simulink model "ElectricalID_ref"  (R2022b)
settings: Solver=FixedStepDiscrete  StartTime=0.0  StopTime=160  FixedStep=0.000005  RelTol=1e-3  EnableMultiTasking=on
settings Model: RequirementInfo={} %GIDa_fe9045fd_0412_4b6e_8206_617cc20e6fde  FPTRunName=Active  Creator=ts  LastModifiedBy=hufnagelde
settings SolverCC: AlgebraicLoopSolver=TrustRegion  PositivePriorityOrder=on  AutoInsertRateTranBlk=on
settings DataIOCC: SaveOutput=off  SignalLogging=off  DSMLogging=off  SaveTime=off
settings OptimizationCC: DefaultParameterBehavior=Inlined  UseDivisionForNetSlopeComputation=on  GainParamInheritBuiltInType=on  UseFloatMulNetSlope=on  DefaultUnderspecifiedDataType=single  UseSpecifiedMinMax=on  InlineInvariantSignals=on  PassReuseOutputArgsAs=Individual arguments  ZeroExternalMemoryAtStartup=off  ZeroInternalMemoryAtStartup=off  NoFixptDivByZeroProtection=on  EfficientFloat2IntCast=on  LifeSpan=1  MaxStackSize=64  OptimizeBlockOrder=speed  DifferentSizesBufferReuse=on  EfficientTunableParamExpr=on
settings DebuggingCC: UnconnectedInputMsg=warning  UnconnectedOutputMsg=warning  UnconnectedLineMsg=warning  BusObjectLabelMismatch=error  AllowSymbolicDim=off  SFUnexpectedBacktrackingDiag=warning  SFNoUnconditionalDefaultTransitionDiag=warning  SFExecutionAtInitializationDiag=none  SFMachineParentedDataDiag=warning  ArithmeticOperatorsInVariantConditions=warning
settings HardwareCC: ProdBitPerPointer=32  ProdBitPerSizeT=32  ProdBitPerPtrDiffT=32  ProdLargestAtomicInteger=Long  ProdLargestAtomicFloat=Double  ProdWordSize=32  ProdLongLongMode=on  ProdHWDeviceType=ARM Compatible->ARM Cortex-R  HardwareBoardFeatureSet=SoCBlockset
settings ModelReferenceCC: EnableRefExpFcnMdlSchedulingChecks=on
settings SFSimCC: SimGenImportedTypeDefs=on  MATLABDynamicMemAlloc=off
settings RTWCC: Description=Embedded Coder  SystemTargetFile=ert.tlc  GenCodeOnly=on  TemplateMakefile=ert_default_tmf  GenerateReport=on  BuildConfiguration=Faster Runs  IncludeHyperlinkInReport=on  LaunchReport=on  GenerateTraceInfo=on  GenerateTraceReport=on  GenerateTraceReportSl=on  GenerateTraceReportSf=on  GenerateTraceReportEml=on  GenerateCodeMetricsReport=on  CheckMdlBeforeBuild=Warning  DLArmComputeVersion=19.05
settings CodeAppCC: ForceParamTrailComments=on  IgnoreCustomStorageClasses=off  OperatorAnnotations=on  SimulinkDataObjDesc=on  SFDataObjDesc=on  MATLABFcnDesc=on  CustomSymbolStrGlobalVar=rt$M$R$N  CustomSymbolStrType=$N$M$R_t  CustomSymbolStrFcn=$N$M$F  CustomSymbolStrMacro=$N$M  InsertBlockDesc=on  StateflowObjectComments=on  MATLABSourceComments=on  EnableCustomComments=on  ReqsInCode=on
settings ERTTargetCC: TargetLangStandard=C99 (ISO)  CodeReplacementLibrary=GNU C99 extensions  MultiwordLength=2048  IncludeMdlTerminateFcn=off  CombineSignalStateStructs=on  SuppressErrorStatus=on  IncludeFileDelimiter=UseQuote  SupportAbsoluteTime=off  CodeInterfacePackaging=Reusable function  SupportNonFinite=off  RemoveResetFunc=off  InlinedParameterPlacement=NonHierarchical  MultiInstanceErrorCode=Warning  RootIOFormat=Part of model data structure  ERTCustomFileTemplate=example_file_process.tlc  GlobalDataDefinition=InSourceFile  GlobalDataReference=InSourceFile  ERTFilePackagingFormat=CompactWithDataFile  SuppressUnreachableDefaultCases=off
settings ConfigComp: CovScope=ReferencedModels  CovSaveName=covdata_rollAP  CovMetricSettings=dcmtrwe  CovHTMLOptions=-sRT=1 -aTS=1 -bRG=1 -bTC=1 -hTR=1 -nFC=0 -scm=1 -bcm=1 -xEv=0  CovSaveCumulativeToWorkspaceVar=on  CovSaveSingleToWorkspaceVar=on  CovCumulativeVarName=covCumulativeData_rollAP  CovReportOnPause=off  CovExternalEMLEnable=off  CovSFcnEnable=off

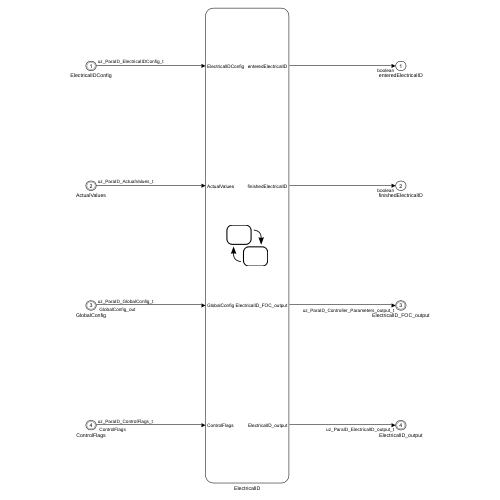
[thumbnail: Simulink's stored preview of the top-level diagram]
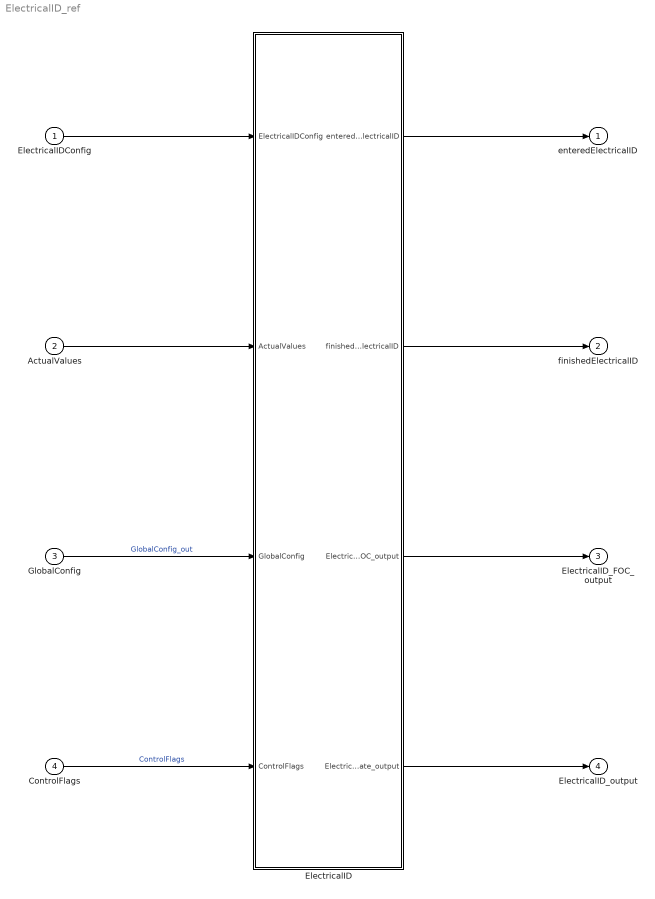
== system ElectricalID_ref ==
  ElectricalIDConfig : Inport  OutDataTypeStr=Bus: uz_ParaID_ElectricalIDConfig_t  PortDimensions=1  SampleTime=[5.0000000000000002e-05,0]  BusOutputAsStruct=on
  ActualValues : Inport  Port=2  OutDataTypeStr=Bus: uz_ParaID_ActualValues_t  PortDimensions=1  SampleTime=[5.0000000000000002e-05,0]  BusOutputAsStruct=on
  GlobalConfig : Inport  Port=3  OutDataTypeStr=Bus: uz_ParaID_GlobalConfig_t  PortDimensions=1  SampleTime=[5.0000000000000002e-05,0]  BusOutputAsStruct=on
  ControlFlags : Inport  Port=4  OutDataTypeStr=Bus: uz_ParaID_ControlFlags_t  PortDimensions=1  SampleTime=[5.0000000000000002e-05,0]  BusOutputAsStruct=on
  ElectricalID : Stateflow chart
  enteredElectricalID : Outport  OutDataTypeStr=boolean  PortDimensions=1  SampleTime=[5.0000000000000002e-05,0]
  finishedElectricalID : Outport  Port=2  OutDataTypeStr=boolean  PortDimensions=1  SampleTime=[5.0000000000000002e-05,0]
  ElectricalID_FOC_output : Outport  Port=3  OutDataTypeStr=Bus: uz_ParaID_Controller_Parameters_output_t  PortDimensions=1  SampleTime=[5.0000000000000002e-05,0]  BusOutputAsStruct=on
  ElectricalID_output : Outport  Port=4  OutDataTypeStr=Bus: uz_ParaID_ElectricalID_output_t  PortDimensions=1  SampleTime=[5.0000000000000002e-05,0]  BusOutputAsStruct=on
  wires:
  ElectricalIDConfig/1 -> ElectricalID/1(ElectricalIDConfig)
  ActualValues/1 -> ElectricalID/2(ActualValues)
  GlobalConfig/1 -> ElectricalID/3(GlobalConfig)  "GlobalConfig_out"
  ControlFlags/1 -> ElectricalID/4(ControlFlags)  "ControlFlags"
  ElectricalID/1(enteredElectricalID) -> enteredElectricalID/1
  ElectricalID/2(finishedElectricalID) -> finishedElectricalID/1
  ElectricalID/3(ElectricalID_FOC_output) -> ElectricalID_FOC_output/1
  ElectricalID/4(ElectricalID_state_output) -> ElectricalID_output/1

== stateflow chart ElectricalID_ref/ElectricalID ==
  settings: updateMethod=DISCRETE  sampleTime=1/d_f_states
  note: PMSM identification
  state ElectricalID
    entry:
    initParams;
    ElectricalID_FOC_output.activeState = uint16(100);
    enteredElectricalID=boolean(1);
    during:
    state stepResponse_q
      entry:
      ElectricalID_FOC_output.activeState = uint16(142);
      resetParams_LM;
      z = uint16(1);
      ElectricalID_state_output.enable_TriState          = [boolean(1),boolean(0),boolean(0)];
      ElectricalID_state_output.PWM_Switch_0 = single(0);
      counter = uint32(1);
      during:
      ElectricalID_state_output.PWM_Switch_4 = single(DutyCycle);
      if(counter <= 1024)
      if(counter > 1)
      measArray1(counter-1) = ActualValues.I_abc.c;
      if(mod(counter,5) == 0)
      Vstep(z-1) = ActualValues.V_abc.b+ActualValues.V_abc.c;
      z = z + 1;
      end
      counter = counter + 1;
      end
      if(counter == 1)
      counter = counter + 1;
      Vstep(1) = ActualValues.V_abc.c+ActualValues.V_abc.b;
      z = z + 1;
      end
      else
      if(counter == 1025)
      measArray1(counter-1) = ActualValues.I_abc.c;
      Vstep(z-1) = ActualValues.V_abc.b+ActualValues.V_abc.c;
      V0 = mean(Vstep);
      end
      ElectricalID_state_output.PWM_Switch_4 = single(0);
      counter = counter + 1;
      end
      exit:
      ElectricalID_state_output.enable_TriState          = [boolean(0),boolean(0),boolean(0)];
    state evaluate_Turn_DC
      entry:
      ElectricalID_FOC_output.activeState = uint16(110);
      counter = uint32(1);
      omega_register=single(zeros(5,1));
      if(ElectricalIDConfig.dutyCyc > 0.0) %Checks if a manual value for the DutyCycle was set
      DutyCycle = single(ElectricalIDConfig.dutyCyc);
      DC_manual = boolean(1);
      else
      DutyCycle = single(0.01);
      end
      during:
      if(DC_manual == 0); %averages the last 0.1s
      omega_sum=omega_sum+single(ActualValues.omega_m);
      if(mod(counter,uint32(0.1/GlobalConfig.sampleTimeISR))==0)
      RefreshDataRegister;
      omega_register(1,1)=omega_sum*(GlobalConfig.sampleTimeISR/0.1);
      omega_sum=single(0);
      end
      if(mod(counter,uint32(2/GlobalConfig.sampleTimeISR))==0)%after 2s omega will be evaluated
      DutyCycle_mod(abs(omega_register));
      end
      end
      counter = counter + 1;
      TurnMotor;
      exit:
      ElectricalID_state_output.PWM_Switch_0 = single(0);
      ElectricalID_state_output.PWM_Switch_2 = single(0);
      ElectricalID_state_output.PWM_Switch_4 = single(0);
    state alignRotor_d_off2
      entry:counter = uint32(1);
      ElectricalID_FOC_output.activeState = uint16(131);
      during:counter = counter +1;
      exit:
    state measure_psiPM
      entry:
      ElectricalID_FOC_output.activeState = uint16(150);
      ElectricalID_FOC_output.enableFOC_speed = boolean(1);
      ElectricalID_FOC_output.n_ref_FOC = ElectricalIDConfig.n_ref_measurement;
      wait_count = uint32(3/GlobalConfig.sampleTimeISR);
      during:
      if(counter > wait_count && counter < (wait_count+1025))
      measArray1(counter-wait_count) = ActualValues.v_dq.q;
      d(counter-wait_count) = ActualValues.i_dq.q;
      i_est(counter-wait_count) = ActualValues.omega_el;
      end
      if(counter == (wait_count+1025))
      ElectricalID_state_output.PMSM_parameters.Psi_PM_Vs = (mean(measArray1(1:1024))-mean(d(1:1024))*....
      ElectricalID_state_output.PMSM_parameters.R_ph_Ohm)/(mean(i_est(1:1024)));
      end
      counter = counter + 1;
      exit:
      counter = uint32(1);
    state stepResponse		%state 2.0
      entry:
      ElectricalID_FOC_output.activeState = uint16(140);
      counter = uint32(1);
      z = uint16(1);
      during:
      ElectricalID_state_output.PWM_Switch_0 = single(DutyCycle);
      if(counter <= 1024)
      if(counter > 1)
      measArray1(counter-1) = ActualValues.I_abc.a;
      if(mod(counter,5) == 0)
      Vstep(z-1) = ActualValues.V_abc.a;
      z = z + 1;
      end
      counter = counter + 1;
      end
      if(counter == 1)
      counter = counter + 1
      Vstep(1) = ActualValues.V_abc.a;
      z = z + 1;
      end
      else
      if(counter == 1025)
      measArray1(counter-1) = ActualValues.I_abc.a;
      Vstep(z-1) = ActualValues.I_abc.a;
      V0 = mean(Vstep);
      end
      ElectricalID_state_output.PWM_Switch_0 = single(0);
      counter = counter + 1;
      end
      exit:
      ElectricalID_FOC_output.activeState = uint16(22);
    state stop 	%state 10.1
      entry:
      ElectricalID_FOC_output.activeState = uint16(151);
      ElectricalID_FOC_output.n_ref_FOC = single(0);
      ElectricalID_FOC_output.resetIntegrator = boolean(1);
      during:counter = counter +1;
    state rotorInertiaEstimation
      entry:
      ElectricalID_FOC_output.enableFOC_speed = boolean(0);
      ElectricalID_FOC_output.enableFOC_torque = boolean(1);
      counter = uint32(1);
      ElectricalID_FOC_output.resetIntegrator = boolean(0);
      ElectricalID_FOC_output.activeState = uint16(160);
      wait_count = uint32(3/GlobalConfig.sampleTimeISR);
      during:
      ElectricalID_FOC_output.M_ref_FOC = SinusGenerator(ElectricalIDConfig.goertzlTorque,....
      ElectricalIDConfig.goertzlFreq,GlobalConfig.sampleTimeISR);
      if(counter > wait_count && counter < (wait_count+501))
      measArray1(counter-wait_count) = ActualValues.i_dq.q;
      i_est(counter-wait_count) = ActualValues.omega_m;
      end
      counter = counter + 1;
      exit:
      goertzel;
    state alignRotor_d_on
      entry:
      ElectricalID_FOC_output.activeState = uint16(120);
      counter = uint32(1);
      during:
      DutyCycle_filt = single(single(counter)*GlobalConfig.sampleTimeISR*2);
      if(DutyCycle_filt > 1)
      DutyCycle_filt = single(1.0);
      end
      ElectricalID_state_output.PWM_Switch_0 = single(DutyCycle*DutyCycle_filt);
      ElectricalID_state_output.PWM_Switch_2 = single(0);
      ElectricalID_state_output.PWM_Switch_4 = single(0);
      counter  = counter +1;
      exit:
      ElectricalID_state_output.PWM_Switch_0 = single(0);
    state Levenberg_Marquardt_q
      entry:
      ElectricalID_FOC_output.activeState = uint16(143);
      LM_algorithm_Lq;
      ElectricalID_state_output.PMSM_parameters.Lq_Henry = L_est*0.5;
      during:
      exit:
    state alignRotor_d_off
      entry:counter = uint32(1);
      ElectricalID_FOC_output.activeState = uint16(121);
      during:counter  = counter +1;
      exit:
      ElectricalID_state_output.thetaOffset = ActualValues.theta_m;
      DutyCycle=single(0.0);%resets the DC and DC_manual flag, so that for the step-response
      DC_manual=boolean(0);  %a new DC can be entered
    state endState
      entry:
      counter = uint32(1);
      ElectricalID_FOC_output.activeState = uint16(161);
      ElectricalID_FOC_output.resetIntegrator=boolean(1);
      ElectricalID_FOC_output.M_ref_FOC = single(0.0);
      during:
      counter = counter + 1;
    state Levenberg_Marquardt 		%state 3.0
      entry:
      ElectricalID_FOC_output.activeState = uint16(141);
      LM_algorithm;
      % calculate R and L. Considering that all three phases
      % are connected and that a delta connected winding has
      % to be calculated into star connected values, the factor
      % is 2/3 for delta and star connected windings.
      % Therefore Rs and Ld are the values expressed in
      % star connection
      ElectricalID_state_output.PMSM_parameters.R_ph_Ohm = (R_est-R_corr)*2.0/3.0;
      ElectricalID_state_output.PMSM_parameters.Ld_Henry = L_est*2.0/3.0;
      during:
      exit:
    state calculatePIcontroller 	%state6.0
      entry:
      ElectricalID_FOC_output.activeState = uint16(144);
      % calculation according to Gemaßmer KIT
      Kp_id_loc = ElectricalID_state_output.PMSM_parameters.Ld_Henry / (3.0 * GlobalConfig.sampleTimeISR) ;
      Ki_id_loc = ElectricalID_state_output.PMSM_parameters.R_ph_Ohm / (3.0 * GlobalConfig.sampleTimeISR) ;
      Ki_iq_loc = Ki_id_loc;
      if (ElectricalIDConfig.identLq == 1)
      Kp_iq_loc = ElectricalID_state_output.PMSM_parameters.Lq_Henry / (3.0 * GlobalConfig.sampleTimeISR) ;
      elseif (ElectricalIDConfig.identLq == 0)
      ElectricalID_state_output.PMSM_parameters.Lq_Henry = ....
      ElectricalID_state_output.PMSM_parameters.Ld_Henry;
      Kp_iq_loc = Kp_id_loc;
      end
      Kp_n_loc = Kp_iq_loc/(ElectricalID_state_output.PMSM_parameters.Lq_Henry*dampingFactor*....
      GlobalConfig.PMSM_config.polePairs*3.0/2.0*psiOverJ);
      Ki_n_loc = (Kp_iq_loc * Kp_iq_loc)/( ElectricalID_state_output.PMSM_parameters.Lq_Henry *....
      ElectricalID_state_output.PMSM_parameters.Lq_Henry  * dampingFactor * dampingFactor * ....
      dampingFactor * GlobalConfig.PMSM_config.polePairs...
      *3.0/2.0*psiOverJ);
      %Output calculated values
      ElectricalID_FOC_output.Kp_id_out = Kp_id_loc;
      ElectricalID_FOC_output.Ki_id_out = Ki_id_loc;
      ElectricalID_FOC_output.Kp_iq_out = Kp_iq_loc;
      ElectricalID_FOC_output.Ki_iq_out = Ki_iq_loc;
      ElectricalID_FOC_output.Kp_n_out = Kp_n_loc;
      ElectricalID_FOC_output.Ki_n_out = single(Ki_n_loc);
    state findDutyCycle	%Motor must be manually locked via load machine until state 60
      entry:
      ElectricalID_FOC_output.activeState = uint16(130);
      if(ElectricalIDConfig.dutyCyc > 0.0)%Checks if a manual value for the DutyCycle was set
      DutyCycle = single(ElectricalIDConfig.dutyCyc);
      DC_manual = boolean(1);
      else
      DutyCycle = single(0.005);
      end
      counter = uint32(1); %starts with 1, so that the DutyCylce_mod function wont be entered
      %during the fist cycle through the state
      during:
      if(DC_manual == 0 && ia_valid==0)
      ElectricalID_state_output.PWM_Switch_0 = single(DutyCycle);
      if(counter < uint32(0.4/GlobalConfig.sampleTimeISR))
      counter = counter +1;
      elseif(counter >= uint32(0.4/GlobalConfig.sampleTimeISR) &&....
      counter < uint32(0.5/GlobalConfig.sampleTimeISR))
      counter = counter +1;
      ia_sum=ia_sum+single(ActualValues.I_abc.a);
      elseif(counter == uint32(0.5/GlobalConfig.sampleTimeISR))
      DutyCycle_mod(abs(ia_sum*(GlobalConfig.sampleTimeISR/0.1)));
      counter  = uint32(1);
      ia_sum = single(0.0);
      end
      end
      exit:
      ElectricalID_state_output.PWM_Switch_0 = single(0);
    state waitState 	%do nothing
      entry:
      counter = uint32(1);
      ElectricalID_FOC_output.enableFOC_torque= boolean(0);
      ElectricalID_FOC_output.activeState = uint16(170);
      % recalculate speed controller using psiPM and J
      Ki_n_loc =....
      (Kp_iq_loc * Kp_iq_loc * 2.0 * pi * ElectricalID_state_output.PMSM_parameters.J_kg_m_squared) /....
      (dampingFactor * dampingFactor * dampingFactor * ElectricalID_state_output.PMSM_parameters.Lq_Henry....
      *ElectricalID_state_output.PMSM_parameters.Lq_Henry *....
      ElectricalID_state_output.PMSM_parameters.Psi_PM_Vs....
      * ElectricalID_state_output.PMSM_parameters.polePairs * 90.0);
      Kp_n_loc =....
      sqrt((dampingFactor * Ki_n_loc * 2.0 * pi * ElectricalID_state_output.PMSM_parameters.J_kg_m_squared)...
      / (90.0 * ElectricalID_state_output.PMSM_parameters.polePairs *....
      ElectricalID_state_output.PMSM_parameters.Psi_PM_Vs));
      ElectricalID_FOC_output.Kp_n_out = Kp_n_loc;
      ElectricalID_FOC_output.Ki_n_out = Ki_n_loc;
      ElectricalID_state_output.PMSM_parameters.I_max_Ampere = GlobalConfig.PMSM_config.I_max_Ampere;
      during:
      counter = counter + 1;
      exit:
      finishedElectricalID=boolean(1);
      enteredElectricalID=boolean(0);
      reset_FOC_output;
    (default) -> evaluate_Turn_DC
    calculatePIcontroller 	%state6.0 -> measure_psiPM : [GlobalConfig.ACCEPT==1]
    findDutyCycle	%Motor must be manually locked via load machine until state 60 -> alignRotor_d_off2 : [ia_valid==1 ||DC_manual == 1]
    alignRotor_d_off2 -> stepResponse		%state 2.0 : [one_sec_transition_counter == counter]
    measure_psiPM -> stop 	%state 10.1 : [ElectricalID_state_output.PMSM_parameters.Psi_PM_Vs > 0]
    stop 	%state 10.1 -> rotorInertiaEstimation : [one_sec_transition_counter == counter]
    evaluate_Turn_DC -> alignRotor_d_on [order 1] : [om_con==1]
    evaluate_Turn_DC -> alignRotor_d_on [order 2] : [DC_manual == 1]
    Levenberg_Marquardt 		%state 3.0 -> stepResponse_q [order 2] : [GlobalConfig.ACCEPT == 1 ....
        | && ElectricalIDConfig.identLq == 1]
    stepResponse_q -> Levenberg_Marquardt_q : [counter == 1026]
    alignRotor_d_on -> alignRotor_d_off : [one_sec_transition_counter == counter]
    stepResponse		%state 2.0 -> Levenberg_Marquardt 		%state 3.0 : [counter == 1026]
    rotorInertiaEstimation -> endState : [counter == (wait_count+513)]
    Levenberg_Marquardt_q -> calculatePIcontroller 	%state6.0
    alignRotor_d_off -> findDutyCycle	%Motor must be manually locked via load machine until state 60 : [one_sec_transition_counter == counter]
    endState -> waitState 	%do nothing : [one_sec_transition_counter == counter]
    Levenberg_Marquardt 		%state 3.0 -> calculatePIcontroller 	%state6.0 [order 1] : [GlobalConfig.ACCEPT == 1 &&....
        |  ElectricalIDConfig.identLq == 0]
  state Waiting
    entry:
    %wait for activation of
    %ElectricalID
    %donothing
  Waiting -> ElectricalID [order 1] : [ControlFlags.startElectricalID==1 &&....
      |  GlobalConfig.Reset==0 && GlobalConfig.ACCEPT==1]
  (default) -> Waiting
  Waiting -> Waiting [order 2] : [GlobalConfig.Reset==1]
      | {finishedElectricalID=boolean(0);
      | enteredElectricalID=boolean(0);
      | initParams;}
  waitState 	%do nothing -> Waiting : [one_sec_transition_counter == counter]
  ElectricalID -> Waiting : [GlobalConfig.Reset==1 || GlobalConfig.ElectricalID==0 ||....
      |  GlobalConfig.enableParameterID==0]
      | {enteredElectricalID=boolean(0);initParams;}
  data: om_reg_in function_input; Amp function_input; Freq function_input; sampleTime function_input; y function_output; ia_reg_in function_input; n_filt local single size=1 =single(0.0); n_ref_old local single size=1 =single(0.0); repetitionCounter local uint32 size=1 =uint32(0); dutyCycAdj local single size=1 =single(0.0); counter local uint32 size=1; k local single size=1; dp local single size=[2,1]; e local single size=1; e_lm local single size=1; it local uint16 size=1; H local single size=[2,2]; L0 local single size=1; R0 local single size=1; Ndata local uint16 size=1; Nparams local uint16 size=1; n_iters local uint16 size=1; lambda local single size=1; updateJ local boolean size=1; V0 local single size=1; DutyCycle_filt local single size=1 =single(0.0); z local uint16 size=1; R_corr local single size=1; dampingFactor local; psiOverJ local; Kp_n_loc local; Ki_n_loc local; Ki_id_loc local; Kp_id_loc local; Ki_iq_loc local; Kp_iq_loc local; meas_sum local single; omega_register local; omega_sum local; om_con local; ia_valid local; ia_sum local; DC_manual local; J2 local; enteredElectricalID output boolean; finishedElectricalID output; ElectricalIDConfig input Bus: uz_ParaID_ElectricalIDConfig_t; ElectricalID_FOC_output output Bus: uz_ParaID_Controller_Parameters_output_t; ActualValues input Bus: uz_ParaID_ActualValues_t; GlobalConfig input Bus: uz_ParaID_GlobalConfig_t; ControlFlags input Bus: uz_ParaID_ControlFlags_t; R_est local single size=1; L_est local single size=1; d local single size=[2048,1]; i_est local single size=[2048,1]; J local single size=[2048,2]; R_lm local single size=1; L_lm local single size=1; Vstep local single size=205; DutyCycle local single; ElectricalID_state_output output Bus: uz_ParaID_ElectricalID_output_t; wait_count local; measArray1 local single size=1024; one_sec_transition_counter local
  function resetParams_LM:
    | function resetParams_LM
    | 
    | % reset variables
    | measArray1			= single(zeros(1024,1));
    | Vstep               = single(zeros(205,1));
    | 
    | % initialize variables for Levenberg-Marquardt
    | d        			= single(zeros(2048,1));
    | dp      			= single(zeros(2,1));
    | e       			= single(0);
    | e_lm  				= single(0);
    | H 					= single(zeros(2,2));
    | i_est 				= single(zeros(2048,1));
    | it 					= uint16(0);
    | J 					= single(zeros(2048,2));
    | k 					= single(0);
    | L0 					= single(0);
    | L_est   			= single(0);
    | L_lm 				= single(0);
    | Ndata  				= uint16(512);
    | Nparams 			= uint16(2);
    | n_iters 			= uint16(100);
    | R0 					= single(0);
    | R_est 				= single(0);
    | R_lm 				= single(0);
    | V0 					= single(0);
    | lambda  			= single(0.01);
    | updateJ 			= boolean(1);
    | %L_d                 = single(0);
    | %R_s                 = single(0);
    | 
    |  
    | end
  function TurnMotor:
    | function TurnMotor
    | 
    | sineCounter = single(counter);
    | 
    | % rechtslauf
    | ElectricalID_state_output.PWM_Switch_0 = 0.5*DutyCycle*sin(2*pi*8*sineCounter*GlobalConfig.sampleTimeISR+pi/2)+0.5;
    | ElectricalID_state_output.PWM_Switch_2 = 0.5*DutyCycle*sin(2*pi*8*sineCounter*GlobalConfig.sampleTimeISR-2*pi/3+pi/2)+0.5;
    | ElectricalID_state_output.PWM_Switch_4 = 0.5*DutyCycle*sin(2*pi*8*sineCounter*GlobalConfig.sampleTimeISR+2*pi/3+pi/2)+0.5;
    | 
    | 
    | % linkslauf
    | % ElectricalID_output.PWM_Switch_0 = DutyCycle*sin(2*pi*8*sineCounter*GlobalConfig.sampleTimeISR+pi/2);
    | % ElectricalID_output.PWM_Switch_2 = DutyCycle*sin(2*pi*8*sineCounter*GlobalConfig.sampleTimeISR+2*pi/3+pi/2);
    | % ElectricalID_output.PWM_Switch_4 = DutyCycle*sin(2*pi*8*sineCounter*GlobalConfig.sampleTimeISR-2*pi/3+pi/2);
  function RefreshDataRegister:
    | function RefreshDataRegister
    | 
    | m=length(omega_register);
    |     for k= single(0):single(m-2)
    |          omega_register(m-k)=omega_register(m-(k+1));
    |      end
    | end
  function DutyCycle_mod(om_reg_in):
    | function DutyCycle_mod(om_reg_in)
    | mean_om_reg=mean(om_reg_in);
    | %if no manual value for the DutyCycle is set, this function determines, if the rotor is turning above
    | %the stated minimal speed and the oscillation is below
    | %the stated threshold
    | 
    | if(om_con==0)
    |     if(mean_om_reg >(ElectricalIDConfig.min_n_ratio*GlobalConfig.ratSpeed*2*pi)/60)%minimal speed in rad/sec
    |         
    |         %determines if the oscillation is below the stated threshold
    |         %(currently 5% of rated speed)
    |           if((mean_om_reg+(0.05*(GlobalConfig.ratSpeed*2*pi)/60))>=max(om_reg_in)&& ...
    |              (mean_om_reg-(0.05*(GlobalConfig.ratSpeed*2*pi)/60))<=min(om_reg_in)&&min(om_reg_in)~=0)
    |          
    |         om_con=boolean(1);    
    |          else
    |          om_con=boolean(0);
    |          end
    |       else
    |           om_con=boolean(0);
    |     end
    | end
    | if(om_con == 0) 
    |     %Increases the DutyCycle by 1% every 2 seconds, if the motor isn't
    |     %rotating properly
    |     DutyCycle = DutyCycle + 0.01; %Simulation 0.001 | Real 0.01
    | end
    | end
  function goertzel:
    | function goertzel
    | 
    | % goertzel algorithm for J calculation
    | 
    | % calculate momentum from i_q
    | for k=single(1):single(500)
    | d(k) = 1.5*GlobalConfig.PMSM_config.polePairs*ElectricalID_state_output.PMSM_parameters.Psi_PM_Vs*measArray1(k);
    | end
    |  
    | % goertzel
    | ISR_factor = single(0.0001 / GlobalConfig.sampleTimeISR); %Adjusts the k-factor for different ISR frequencys
    | k = single(2.0 / ISR_factor);   % coefficient number of the spectrum (40Hz)
    | N = 500;       % length of input signal
    | 
    | %Precalculation of constants
    | A = 2*pi*k/N;
    | B = 2*cos(A);
    | C = exp(-j*A);
    | %State variables
    | s0 = single(0.0);
    | s1 = single(0.0);
    | s2 = single(0.0);
    | 
    | %Main loop for M
    | for i = 1:N %N multiplications, 2N additions
    | s0 = d(i) +B*s1-s2; %corresponds to (16)
    | s2 = s1;
    | s1 = s0;
    | end
    | 
    | %Finalizing calculations for M
    | s0 = B*s1-s2; %corresponds to (16) with zero input; 1 multiplication and 1 addition
    | Xg = s0-s1*C %corresponds to (17); 4 multiplications and 3 additions
    | 
    | %Reset state variables
    | s0 = single(0.0);
    | s1 = single(0.0);
    | s2 = single(0.0);
    | 
    | %Main loop for omega_m
    | for i = 1:N %N multiplications, 2N additions
    | s0 = i_est(i) +B*s1-s2; %corresponds to (16)
    | s2 = s1;
    | s1 = s0;
    | end
    | 
    | %Finalizing calculations for omega_m
    | s0 = B*s1-s2; %corresponds to (16) with zero input; 1 multiplication and 1 addition
    | Yg = s0-s1*C %corresponds to (17); 4 multiplications and 3 additions
    | 
    | 
    | 
    | % calculate value of transfer function 
    | Gg = Yg/Xg;
    | % calculate J from Gg
    | ElectricalID_state_output.PMSM_parameters.J_kg_m_squared = single(abs(1/(Gg*j*2*pi*40))); %without damping
  function y = SinusGenerator(Amp, Freq, sampleTime):
    | function y = SinusGenerator(Amp, Freq, sampleTime)
    | %#codegen
    | 
    | persistent sineCounter;
    | 
    | if isempty(sineCounter)
    |     sineCounter = uint32(0); %initialize
    |     u = single(0);
    | end
    |     u = single(Amp*sin(2*pi*single(Freq)*single(sineCounter)*sampleTime));
    |     sineCounter = sineCounter + 1;
    |     if(sineCounter == uint32(1/(single(Freq)*sampleTime)))
    |         sineCounter = uint32(0);
    |     end
    |    
    | 
    | y = single(u);
  function LM_algorithm_Lq:
    | function LM_algorithm_Lq
    |    
    |     
    | % Startwerte Festlegen
    | %V0 = V_s;                           % Spannungssprung in Volt
    | R0 = single(0.001000);              % Widerstand in Ohm (0.01 ... 40 Ohm)
    | L0 = single(0.000005);              % Induktivitaet in Henry (0.05mH ... 50 mH)
    | 
    | R_est   = R0;
    | L_est   = L0;
    | %#codegen
    | 
    | % Levenberg-Marquardt Curve Fitting
    | 
    | % i_input(Stromwerte) -> Stromwerte in A !!!
    | 
    | % Mathematische Grundlagen mit Symbolic Toolbox erstellen
    |     %syms U R L t i real;                   %Symbolische Variablen erstellen
    |     %f = U/R*(1-exp(-R*t/L))                %Modellfunktion (Laden einer Spule)
    |     %d = i-f;                               %Fehler d = Messung - Modell
    |     %Jsym = jacobian(d,[R L])               %Jacobi-Matrix des Fehlers (Ableitungen nach den Parametern R und L)                  
    | 
    |     
    |     % Parameterbestimmung durch Iteration
    |     for it=uint16(1):n_iters
    |         if updateJ == 1
    |             % Jacobi-Matrix mit aktuellem Parametersatz berechnen
    |             for k=single(1):single(1024)
    |              J(k,:) = [- (V0*(exp(-(R_est*(k-1)*GlobalConfig.sampleTimeISR)/L_est)....
    |                  - 1))/R_est^2 - (V0*(k-1)*GlobalConfig.sampleTimeISR*exp....
    |                  (-(R_est*(k-1)*GlobalConfig.sampleTimeISR)/L_est))/(L_est*R_est)....
    |                  , (V0*(k-1)*GlobalConfig.sampleTimeISR*exp(-(R_est*(k-1)*....
    |                  GlobalConfig.sampleTimeISR)/L_est))/L_est^2];
    |             end
    |             % Modellfunktion mit aktuellem Parametersatz berechnen
    |             for k=single(1):single(1024)
    |             i_est(k) = V0/R_est*(1-exp(-R_est*((k-1)*GlobalConfig.sampleTimeISR)/L_est));
    |             end
    |             % Fehler zwischen Messdaten und Modellfunktionswerten berechnen
    |             d(1:1024) = measArray1(1:1024)-i_est(1:1024);
    |             % Approximierte Hesse-Matrix berechnen
    |             H = J(1:1024,:)'*J(1:1024,:);
    |             if it==1
    |                 e = dot(d,d);           % Fehlerquadrat berechnen
    |             end
    |         end
    |         
    |         % Daempfungsfaktor lambda auf Hesse-Matrix anwenden
    |         H(1,1) = H(1,1) + lambda;
    |         H(2,2)=H(2,2)+lambda;
    |         
    |         % Neue Paramterschaetzung berechnen
    |         dp = -inv(H)*(J(1:1024,:)'*d(1:1024));
    |         R_lm = R_est + dp(1);
    |         L_lm = L_est + dp(2);
    |         
    |         % Modellfunktion mit neuem Parametersatz berechnen
    |         for k=single(1):single(1024)
    |         i_est(k) = V0/R_lm*(1-exp(-R_lm*((k-1)*GlobalConfig.sampleTimeISR)/L_lm));
    |         end
    |         % Fehler und Fehlerquadrate neu berechnen
    |         d(1:1024) = measArray1(1:1024) - i_est(1:1024);
    |         e_lm = dot(d(1:1024),d(1:1024));
    |         
    |         % Fallunterscheidung ob Fehler groesser oder kleiner geworden ist
    |         if e_lm < e
    |             lambda = lambda/10;
    |             R_est = R_lm;
    |             L_est = L_lm;
    |             e = e_lm;
    |             updateJ = boolean(1);
    |         else
    |             updateJ = boolean(0);
    |             lambda = lambda*10;
    |         end
    |     end
  function LM_algorithm:
    | function LM_algorithm
    |    
    |     
    | % Startwerte Festlegen
    | %V0 = V_s;                           % Spannungssprung in Volt
    | R0 = single(0.001000);              % Widerstand in Ohm (0.01 ... 40 Ohm)
    | L0 = single(0.000005);              % Induktivitaet in Henry (0.05mH ... 50 mH)
    | 
    | R_est   = R0;
    | L_est   = L0;
    | %#codegen
    | 
    | % Levenberg-Marquardt Curve Fitting
    | 
    | % i_input(Stromwerte) -> Stromwerte in A !!!
    | 
    | % Mathematische Grundlagen mit Symbolic Toolbox erstellen
    |     %syms U R L t i real;                   %Symbolische Variablen erstellen
    |     %f = U/R*(1-exp(-R*t/L))                %Modellfunktion (Laden einer Spule)
    |     %d = i-f;                               %Fehler d = Messung - Modell
    |     %Jsym = jacobian(d,[R L])               %Jacobi-Matrix des Fehlers (Ableitungen nach den Parametern R und L)                  
    | 
    |     
    |     % Parameterbestimmung durch Iteration
    |     for it=uint16(1):n_iters
    |         if updateJ == 1
    |             % Jacobi-Matrix mit aktuellem Parametersatz berechnen
    |             for k=single(1):single(1024)
    |              J(k,:) = [- (V0*(exp(-(R_est*(k-1)*GlobalConfig.sampleTimeISR)/L_est)....
    |                  - 1))/R_est^2 - (V0*(k-1)*GlobalConfig.sampleTimeISR*exp....
    |                  (-(R_est*(k-1)*GlobalConfig.sampleTimeISR)/L_est))/(L_est*R_est)....
    |                  , (V0*(k-1)*GlobalConfig.sampleTimeISR*exp(-(R_est*(k-1)*....
    |                  GlobalConfig.sampleTimeISR)/L_est))/L_est^2];
    |             end
    |             % Modellfunktion mit aktuellem Parametersatz berechnen
    |             for k=single(1):single(1024)
    |             i_est(k) = V0/R_est*(1-exp(-R_est*((k-1)*GlobalConfig.sampleTimeISR)/L_est));
    |             end
    |             % Fehler zwischen Messdaten und Modellfunktionswerten berechnen
    |             d(1:1024) = measArray1(1:1024)-i_est(1:1024);
    |             % Approximierte Hesse-Matrix berechnen
    |             H = J(1:1024,:)'*J(1:1024,:);
    |             if it==1
    |                 e = dot(d,d);           % Fehlerquadrat berechnen
    |             end
    |         end
    |         
    |         % Daempfungsfaktor lambda auf Hesse-Matrix anwenden
    |         H(1,1) = H(1,1) + lambda;
    |         H(2,2)=H(2,2)+lambda;
    |         
    |         % Neue Paramterschaetzung berechnen
    |         dp = -inv(H)*(J(1:1024,:)'*d(1:1024));
    |         R_lm = R_est + dp(1);
    |         L_lm = L_est + dp(2);
    |         
    |         % Modellfunktion mit neuem Parametersatz berechnen
    |         for k=single(1):single(1024)
    |         i_est(k) = V0/R_lm*(1-exp(-R_lm*((k-1)*GlobalConfig.sampleTimeISR)/L_lm));
    |         end
    |         % Fehler und Fehlerquadrate neu berechnen
    |         d(1:1024) = measArray1(1:1024) - i_est(1:1024);
    |         e_lm = dot(d(1:1024),d(1:1024));
    |         
    |         % Fallunterscheidung ob Fehler groesser oder kleiner geworden ist
    |         if e_lm < e
    |             lambda = lambda/10;
    |             R_est = R_lm;
    |             L_est = L_lm;
    |             e = e_lm;
    |             updateJ = boolean(1);
    |         else
    |             updateJ = boolean(0);
    |             lambda = lambda*10;
    |         end
    |     end
  function DutyCycle_mod(ia_reg_in):
    | function DutyCycle_mod(ia_reg_in)
    | 
    | mean_ia_reg=mean(ia_reg_in);
    | %determines if the mean value is below the step-response current limit
    | if(mean_ia_reg < 0.5*GlobalConfig.ratCurrent)%Current limit for step response  
    | 	ia_valid=boolean(0);    
    | else
    |     ia_valid=boolean(1);
    | end
    |    
    | if(ia_valid == 0)
    | 	%Increases the DutyCycle by 0.5% every 0.5 second, if the step response
    | 	%is below the current limit
    | 	DutyCycle = DutyCycle + 0.005; %Simulation 0.001 | Real 0.005
    | end
    | end
  function initParams:
    | function initParams
    | 
    | %This is used instead of "after(1.0,sec) to ensure the same transition time
    | %independelty of the sampletime in the c-code
    | one_sec_transition_counter = uint32(1/GlobalConfig.sampleTimeISR);
    | % initialize variables
    | Ki_n_loc            = single(0.0);
    | Kp_n_loc            = single(0.0);
    | n_filt              = single(0.0);
    | n_ref_old           = single(0.0);
    | repetitionCounter   = uint32(0);
    | dutyCycAdj          = single(0.0);
    | counter 			= uint32(1);
    | Kp_iq_loc           = single(0.0);
    | Ki_iq_loc           = single(0.0);
    | Kp_id_loc           = single(0.0);
    | Ki_id_loc           = single(0.0);
    | DutyCycle_filt      = single(0.0);
    | measArray1			= single(zeros(1024,1));
    | meas_sum            = single(zeros(2,1));%used for Friction Id
    | J2                  = single(zeros(256,5));
    | thetaOffset         = single(0.0);
    | Vstep               = single(zeros(205,1));
    | DutyCycle           = single(0.0);
    | omega_sum           = single(0);
    | om_con              = boolean(0);
    | ia_sum              = single(0);
    | ia_valid            = boolean(0);
    | DC_manual           = boolean(0);
    | 
    | %Outputs
    | ElectricalID_FOC_output.Ki_n_out                    = single(0.0);
    | ElectricalID_FOC_output.Ki_iq_out                   = single(0.0);
    | ElectricalID_FOC_output.Ki_id_out                   = single(0.0);
    | ElectricalID_FOC_output.Kp_n_out                    = single(0.0);
    | ElectricalID_FOC_output.Kp_iq_out                   = single(0.0);
    | ElectricalID_FOC_output.Kp_id_out                   = single(0.0);
    | ElectricalID_FOC_output.n_ref_FOC                   = single(0.0);
    | ElectricalID_FOC_output.M_ref_FOC                   = single(0.0);
    | ElectricalID_FOC_output.i_dq_ref.d                  = single(0.0);
    | ElectricalID_FOC_output.i_dq_ref.q                  = single(0.0);
    | ElectricalID_FOC_output.i_dq_ref.zero               = single(0.0);
    | ElectricalID_FOC_output.enableFOC_speed             = boolean(0);
    | ElectricalID_FOC_output.enableFOC_current           = boolean(0);
    | ElectricalID_FOC_output.enableFOC_torque            = boolean(0);
    | ElectricalID_FOC_output.resetIntegrator             = boolean(0);
    | ElectricalID_FOC_output.activeState                 = uint16(0);
    | finishedElectricalID= boolean(0);
    | 
    | ElectricalID_state_output.PWM_Switch_0                        = single(0.0);
    | ElectricalID_state_output.PWM_Switch_2                        = single(0.0);
    | ElectricalID_state_output.PWM_Switch_4                        = single(0.0);
    | ElectricalID_state_output.enable_TriState                     = boolean(zeros(1,3)); %0 = TriState off, 1 = TriState on   
    | ElectricalID_FOC_output.activeState                     = uint16(0);
    | ElectricalID_state_output.thetaOffset                         = single(0.0);
    | ElectricalID_state_output.PMSM_parameters.R_ph_Ohm            = single(0.0);
    | ElectricalID_state_output.PMSM_parameters.Ld_Henry            = single(0.0);
    | ElectricalID_state_output.PMSM_parameters.Lq_Henry            = single(0.0);
    | ElectricalID_state_output.PMSM_parameters.Psi_PM_Vs           = single(0.0);
    | ElectricalID_state_output.PMSM_parameters.polePairs           = GlobalConfig.PMSM_config.polePairs;
    | ElectricalID_state_output.PMSM_parameters.J_kg_m_squared      = single(0.0);
    | enteredElectricalID                                     = boolean(0);
    | 
    | % initialize variables for Levenberg-Marquardt
    | d        			= single(zeros(2048,1));
    | dp      			= single(zeros(2,1));
    | e       			= single(0);
    | e_lm  				= single(0);
    | H 					= single(zeros(2,2));
    | i_est 				= single(zeros(2048,1));
    | it 					= uint16(0);
    | J 					= single(zeros(2048,2));
    | k 					= single(0);
    | L0 					= single(0);
    | L_est   			= single(0);
    | L_lm 				= single(0);
    | Ndata  				= uint16(512);
    | Nparams 			= uint16(2);
    | n_iters 			= uint16(100);
    | R0 					= single(0);
    | R_est 				= single(0);
    | R_lm 				= single(0);
    | V0 					= single(0);
    | lambda  			= single(0.01);
    | updateJ 			= boolean(1);
    | 
    | % initialize varaibles for PMSM parameters
    | R_corr              = single(0.000); %0.060
    | 
    | % variables for controller calculation
    | dampingFactor           = single(10.0);
    | psiOverJ                = single(1000);
    | 
    | end
  function reset_FOC_output:
    | function reset_FOC_output
    | 
    | %Outputs
    | ElectricalID_FOC_output.n_ref_FOC           = single(0.0);
    | ElectricalID_FOC_output.M_ref_FOC           = single(0.0);
    | ElectricalID_FOC_output.i_dq_ref.d          = single(0.0);
    | ElectricalID_FOC_output.i_dq_ref.q          = single(0.0);
    | ElectricalID_FOC_output.i_dq_ref.zero       = single(0.0);
    | ElectricalID_FOC_output.enableFOC_speed     = boolean(0);
    | ElectricalID_FOC_output.enableFOC_current   = boolean(0);
    | ElectricalID_FOC_output.enableFOC_torque    = boolean(0);
    | ElectricalID_FOC_output.resetIntegrator     = boolean(0);
    | ElectricalID_FOC_output.activeState         = uint16(0);
    | ElectricalID_FOC_output.Kp_id_out              = single(Kp_id_loc);
    | ElectricalID_FOC_output.Kp_iq_out              = single(Kp_iq_loc);
    | ElectricalID_FOC_output.Kp_n_out               = single(Kp_n_loc);
    | ElectricalID_FOC_output.Ki_id_out              = single(Ki_id_loc);
    | ElectricalID_FOC_output.Ki_iq_out              = single(Ki_iq_loc);
    | ElectricalID_FOC_output.Ki_n_out               = single(Ki_n_loc);
    | end
